simulink model "manip_model"  (R2021b)
settings: Solver=VariableStepAuto  StartTime=0.0  StopTime=30  RelTol=1e-3
values from neighbouring files (symbols this model uses):
  n = str2num(answer{1})    [main.m]    (also in manip_animation.m = numel(q))
libraries: slpidlib x1, cstblocks x1
settings Model: Creator=User  LastModifiedBy=User

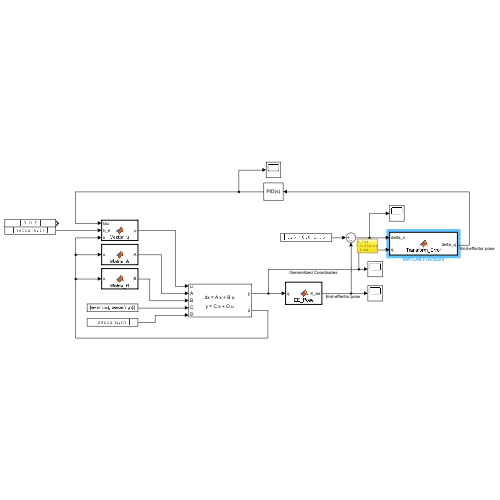
[thumbnail: Simulink's stored preview of the top-level diagram]
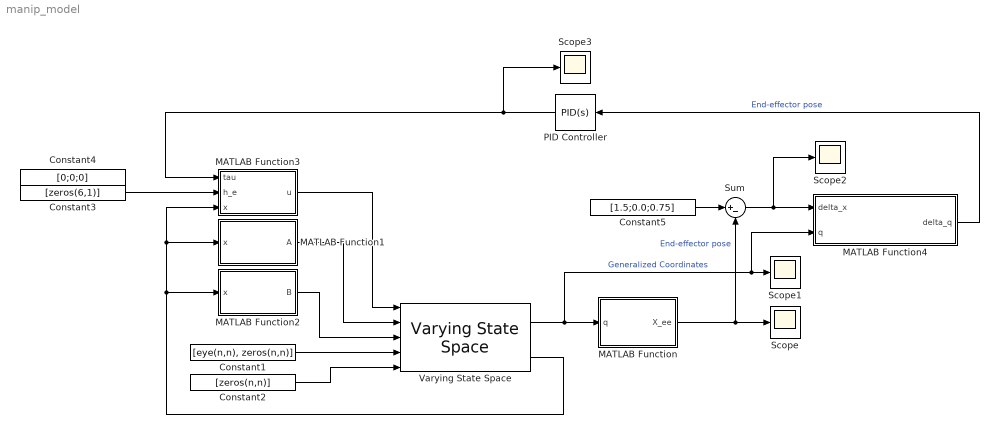
== system manip_model ==
  Constant1 : Constant  Value=[eye(n,n), zeros(n,n)]
  Constant2 : Constant  Value=[zeros(n,n)]
  Constant3 : Constant  Value=[zeros(6,1)]
  Constant4 : Constant  Value=[0;0;0]
  Constant5 : Constant  Value=[1.5;0.0;0.75]
  MATLAB Function : MATLAB Function  TreatAsAtomicUnit=on
  MATLAB Function1 : MATLAB Function  TreatAsAtomicUnit=on
  MATLAB Function2 : MATLAB Function  TreatAsAtomicUnit=on
  MATLAB Function3 : MATLAB Function  TreatAsAtomicUnit=on
  MATLAB Function4 : MATLAB Function  TreatAsAtomicUnit=on
  PID Controller : slpidlib/PID Controller  Controller=PID  Form=Parallel  TimeDomain=Continuous-time  UseExternalTs=off  SampleTime=-1  IntegratorMethod=Forward Euler  FilterMethod=Forward Euler  ControllerParametersSource=internal  P=0.0001  I=10  D=0  UseFilter=on  N=100  TunerSelectOption=Transfer Function Based (PID Tuner App)  InitialConditionSource=internal  InitialConditionForIntegrator=0  InitialConditionForFilter=0  DifferentiatorICPrevScaledInput=0  ExternalReset=none  TrackingMode=off  Kt=1  LimitOutput=off  SatLimitsSource=internal  UpperSaturationLimit=inf  LowerSaturationLimit=-inf  LinearizeAsGain=on  AntiWindupMode=none  Kb=1  POutMin=[]  POutMax=[]  IOutMin=[]  IOutMax=[]  DOutMin=[]  DOutMax=[]  NOutMin=[]  NOutMax=[]  SumOutMin=[]  SumOutMax=[]  SaturationOutMin=[]  SaturationOutMax=[]  PParamMin=[]  PParamMax=[]  IParamMin=[]  IParamMax=[]  DParamMin=[]  DParamMax=[]  NParamMin=[]  NParamMax=[]  KbParamMin=[]  KbParamMax=[]  KtParamMin=[]  KtParamMax=[]  KbOutMin=[]  KbOutMax=[]  KtOutMin=[]  KtOutMax=[]  IntegratorOutMin=[]  IntegratorOutMax=[]  FilterOutMin=[]  FilterOutMax=[]  SumI1OutMin=[]  SumI1OutMax=[]  SumI2OutMin=[]  SumI2OutMax=[]  SumI3OutMin=[]  SumI3OutMax=[]  SumI4OutMin=[]  SumI4OutMax=[]  SumDOutMin=[]  SumDOutMax=[]  DifferentiatorOutMin=[]  DifferentiatorOutMax=[]  FilterDiffOutCoefMin=[]  FilterDiffOutCoefMax=[]  ReciprocalOutMin=[]  ReciprocalOutMax=[]  SumDenOutMin=[]  SumDenOutMax=[]  SumNumOutMin=[]  SumNumOutMax=[]  DivideOutMin=[]  DivideOutMax=[]  UdiffTsProdOutMin=[]  UdiffTsProdOutMax=[]  NTsProdOutMin=[]  NTsProdOutMax=[]  UintegralTsProdOutMin=[]  UintegralTsProdOutMax=[]  UngainTsProdOutMin=[]  UngainTsProdOutMax=[]  IntegratorContinuousStateAttributes=''  IntegratorStateMustResolveToSignalObject=off  IntegratorRTWStateStorageClass=Auto  FilterContinuousStateAttributes=''  FilterStateMustResolveToSignalObject=off  FilterRTWStateStorageClass=Auto  ParallelPVariant=InternalParameters  IdealPVariant=Disabled  IVariant=InternalParameters  DVariant=InternalParameters  IntegratorVariant=Continuous  SatVariant=Disabled  AWVariant=Passthrough  PCopyVariant=Disabled  TRVariant=Disabled  FdbkBlocksVariant=Forward  IdealPFdbkVariant=Disabled  SatFdbkVariant=Disabled  DerivativeFilterVariant=ContFilter  NVariant=InternalParameters  NCopyVariant=Disabled  FilterICVariant=InternalICsFilter  IntegratorICVariant=InternalICs  ExternalResetVariant=Disabled  TRSumVariant=Passthrough  SumFdbkVariant=Disabled  SumVariant=Sum_PID  TsampFilterVariant=InternalTs  TsampNgainVariant=Passthrough  TsampIntegralVariant=Passthrough  ExternalSaturationOutDataTypeStr=Inherit: Same as second input
  Scope{,1..3} (4 alike) : Scope
  Sum : Sum  Inputs=|+-
  Varying State Space : cstblocks/Linear Parameter Varying/Varying State Space  x0=zeros(2*n, 1)  xNames=''  OutputX=on  OutputDX=off
  wires:
  MATLAB Function/1(X_ee) -> Sum/2, Scope/1  "End-effector pose"
  MATLAB Function1/1(A) -> Varying State Space/2
  MATLAB Function2/1(B) -> Varying State Space/3
  Constant1/1 -> Varying State Space/4
  Constant2/1 -> Varying State Space/5
  Varying State Space/1 -> MATLAB Function4/2(q), Scope1/1, MATLAB Function/1(q)  "Generalized Coordinates"
  Varying State Space/2 -> MATLAB Function3/3(x), MATLAB Function1/1(x), MATLAB Function2/1(x)
  Constant3/1 -> MATLAB Function3/2(h_e)
  MATLAB Function3/1(u) -> Varying State Space/1
  Constant5/1 -> Sum/1
  Sum/1 -> Scope2/1, MATLAB Function4/1(delta_x)
  MATLAB Function4/1(delta_q) -> PID Controller/1  "End-effector pose"
  PID Controller/1 -> Scope3/1, MATLAB Function3/1(tau)

== matlab function manip_model/MATLAB Function ==
  data: q input; X_ee output size=[3 1]
function X_ee = EE_Pose(q)

X_ee = get_X_ee(q);

== matlab function manip_model/MATLAB Function2 ==
  data: x input size=[2*n 1]; B output size=[2*n n]
function B = Matrix_B(x)
    n = numel(x)/2;

    B = [zeros(n); get_M(x(1:n))^-1];

== matlab function manip_model/MATLAB Function3 ==
  data: tau input size=[n 1]; h_e input size=[6 1]; x input size=[2*n 1]; u output size=[n 1]
function u = Vector_u(tau,h_e,x)
n = numel(x)/2;

u = -get_g(x(1:n)) + get_J_ee(x(1:n))'*h_e + tau;

== matlab function manip_model/MATLAB Function4 ==
  data: delta_x input size=[3 1]; q input; delta_q output size=[n 1]
function delta_q = Transform_Error(delta_x, q)

    %delta_q =  get_Jw_ee(q)' * delta_x;
    delta_q =  pinv(get_Jw_ee(q)) * delta_x;

== matlab function manip_model/MATLAB Function1 ==
  data: x input size=[2*n 1]; A output size=[2*n 2*n]
function A = Matrix_A(x)
n = numel(x)/2;

A = [zeros(n), eye(n);
     zeros(n), -get_M(x(1:n))^-1 * ( get_C(x) + get_D(x) )];
